simulink model "sudarshan_simulink1"  (R2021b)
settings: Solver=VariableStepAuto  StartTime=0.0  StopTime=10  RelTol=1e-3
libraries: simulink x1
settings Model: Creator=exam  LastModifiedBy=year2

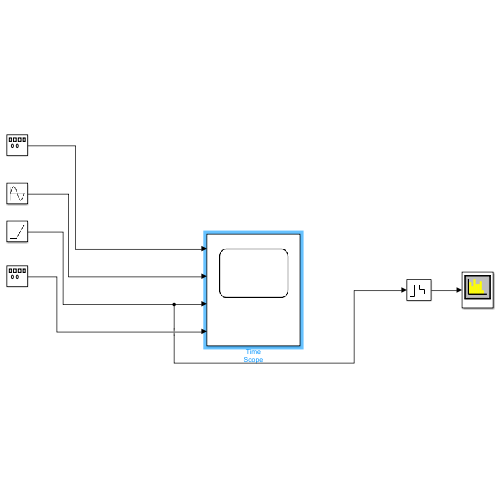
[thumbnail: Simulink's stored preview of the top-level diagram]
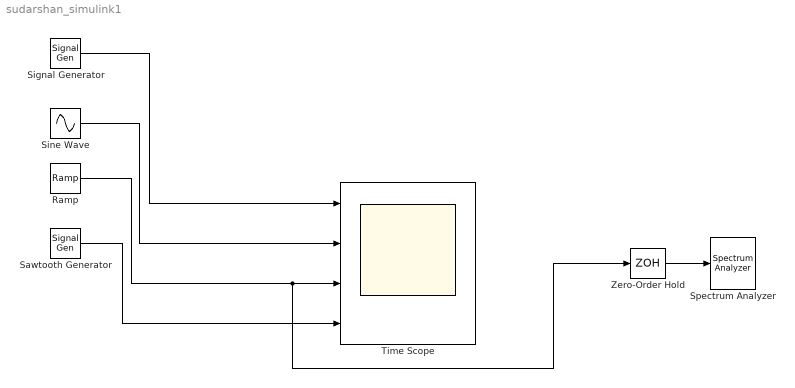
== system sudarshan_simulink1 ==
  Ramp : simulink/Sources/Ramp  slope=1  start=0  InitialOutput=0
  Sawtooth Generator : SignalGenerator  WaveForm=sawtooth  Units=rad/sec
  Signal Generator : SignalGenerator  Units=rad/sec
  Sine Wave : Sin  SampleTime=0
  Spectrum Analyzer : SpectrumAnalyzer
  Time Scope : Scope  NumInputPorts=4
  Zero-Order Hold : ZeroOrderHold  SampleTime=-1
  wires:
  Signal Generator/1 -> Time Scope/1
  Sawtooth Generator/1 -> Time Scope/4
  Sine Wave/1 -> Time Scope/2
  Ramp/1 -> Zero-Order Hold/1, Time Scope/3
  Zero-Order Hold/1 -> Spectrum Analyzer/1
